simulink model "untitled"  (Simulink 9.0)
settings: Solver=ode5  StartTime=0.0  StopTime=10.0  FixedStep=0.001  RelTol=1e-3
undefined symbols (not defined in the file): g, k, k1, k2, l, L1, L2, m
settings Model: Creator=HpZ-R  LastModifiedBy=HpZ-R
settings DataIOCC: SaveFormat=Dataset
settings OptimizationCC: LifeSpan=auto
settings DebuggingCC: UnderspecifiedInitializationDetection=Simplified  MergeDetectMultiDrivingBlocksExec=error  SFUnexpectedBacktrackingDiag=error  SFNoUnconditionalDefaultTransitionDiag=error  SFExecutionAtInitializationDiag=warning
settings HardwareCC: ProdBitPerPointer=64  ProdBitPerSizeT=64  ProdBitPerPtrDiffT=64  ProdLargestAtomicFloat=Float  ProdIntDivRoundTo=Zero  ProdEndianess=LittleEndian  ProdWordSize=64  ProdHWDeviceType=Intel->x86-64 (Windows64)
settings ModelReferenceCC: PropagateSignalLabelsOutOfModel=on
settings CodeAppCC: StateflowObjectComments=off
settings GRTTargetCC: TargetLangStandard=C99 (ISO)
settings ConfigComp: CovMetricSettings=dwe  CovHtmlReporting=off  CovSaveCumulativeToWorkspaceVar=off  CovSaveSingleToWorkspaceVar=off  CovExternalEMLEnable=on

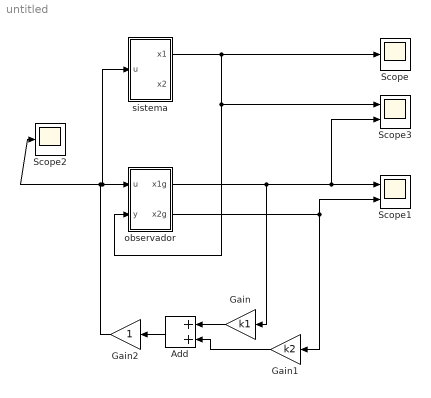
== system untitled ==
  Add : Sum
  Gain : Gain  Gain=k1
  Gain1 : Gain  Gain=k2
  Gain2 : Gain
  Scope : Scope
  Scope1 : Scope  NumInputPorts=2
  Scope2 : Scope
  Scope3 : Scope  NumInputPorts=2
  observador : Subsystem
  sistema : Subsystem
  wires:
  sistema/1("x1 ") -> Scope3/1, observador/2(y), Scope/1
  Add/1 -> Gain2/1
  observador/1(x1g) -> Gain/1, Scope3/2, Scope1/1
  observador/2(x2g) -> Scope1/2, Gain1/1
  Gain/1 -> Add/1
  Gain1/1 -> Add/2
  Gain2/1 -> sistema/1(u), observador/1(u), Scope2/1

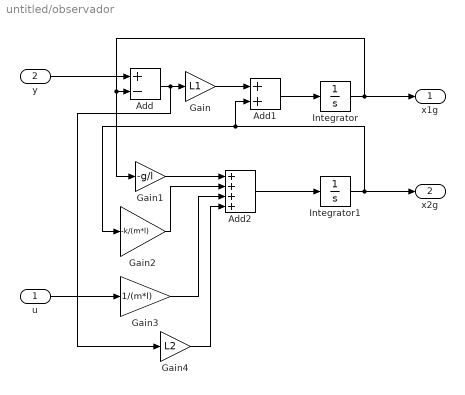
== system untitled/observador ==
  u : Inport
  y : Inport  Port=2
  Add : Sum  Inputs=+-
  Add1 : Sum
  Add2 : Sum  Inputs=++++
  Gain : Gain  Gain=L1
  Gain1 : Gain  Gain=-g/l
  Gain2 : Gain  Gain=-k/(m*l)
  Gain3 : Gain  Gain=1/(m*l)
  Gain4 : Gain  Gain=L2
  Integrator : Integrator
  Integrator1 : Integrator
  x1g : Outport
  x2g : Outport  Port=2
  wires:
  Integrator1/1 -> Add1/2, Gain2/1, x2g/1
  Gain4/1 -> Add2/4
  Gain/1 -> Add1/1
  Add/1 -> Gain4/1, Gain/1
  Add1/1 -> Integrator/1
  Integrator/1 -> x1g/1, Add/2, Gain1/1
  Gain2/1 -> Add2/2
  Gain3/1 -> Add2/3
  y/1 -> Add/1
  u/1 -> Gain3/1
  Gain1/1 -> Add2/1
  Add2/1 -> Integrator1/1

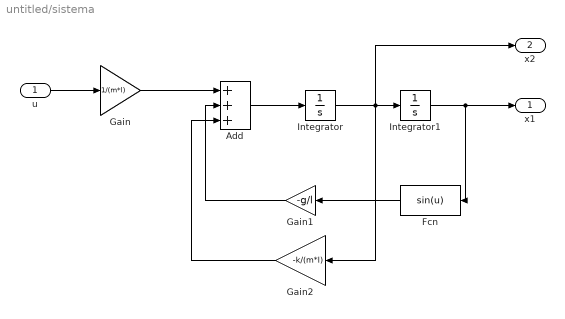
== system untitled/sistema ==
  u : Inport
  Add : Sum  Inputs=+++
  Fcn : Fcn  Expr=sin(u)
  Gain : Gain  Gain=1/(m*l)
  Gain1 : Gain  Gain=-g/l
  Gain2 : Gain  Gain=-k/(m*l)
  Integrator : Integrator
  Integrator1 : Integrator  InitialCondition=pi/2
  "x1 " : Outport
  x2 : Outport  Port=2
  wires:
  Integrator/1 -> x2/1, Gain2/1, Integrator1/1
  Gain/1 -> Add/1
  Integrator1/1 -> "x1 "/1, Fcn/1
  u/1 -> Gain/1
  Add/1 -> Integrator/1
  Gain1/1 -> Add/2
  Gain2/1 -> Add/3
  Fcn/1 -> Gain1/1
